simulink model "SegOrdem"  (R2015a)
settings: Solver=ode45  StartTime=0.0  StopTime=60  FixedStep=0.00001  RelTol=1e-5
settings Model: Creator=user  LastModifiedBy=user
settings SolverCC: ZeroCrossAlgorithm=Adaptive
settings DebuggingCC: UnderspecifiedInitializationDetection=Classic

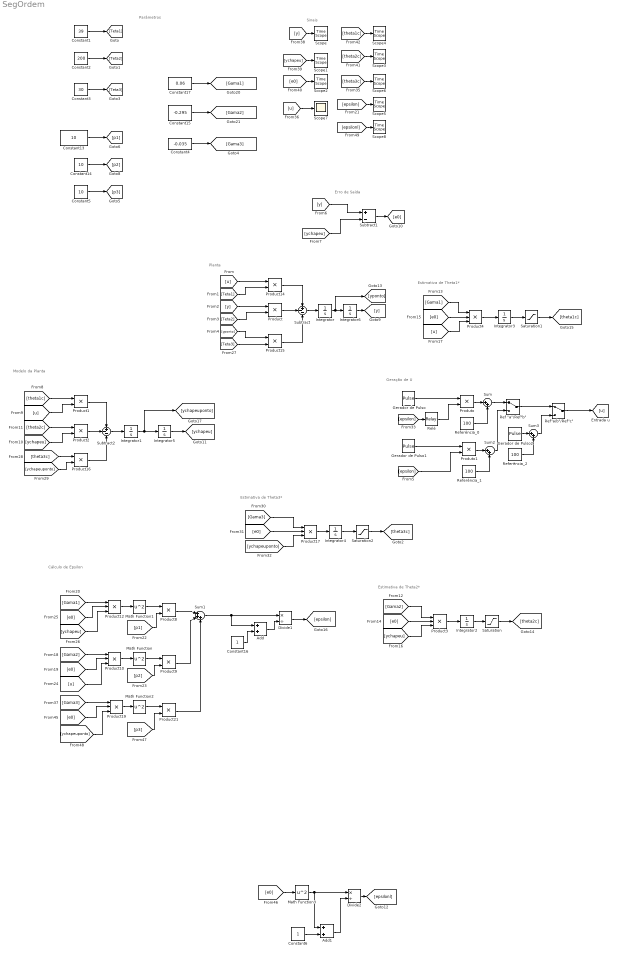
== system SegOrdem ==
  note: Cálculo de Epsilon
  note: Estimativa de Theta1*
  note: Estimativa de Theta2*
  note: Modelo da Planta
  note: Erro de Saída
  note: Parâmetros
  note: Sinais
  note: Estimativa de Theta3*
  note: Planta
  note: Geração de U
  Add : Sum  AccumDataTypeStr=double
  Add1 : Sum  AccumDataTypeStr=double
  Constant1 : Constant  Value=39
  Constant13 : Constant  Value=10
  Constant14 : Constant  Value=10
  Constant15 : Constant  Value=-0.295
  Constant16 : Constant
  Constant17 : Constant  Value=0.06
  Constant2 : Constant  Value=200
  Constant3 : Constant  Value=30
  Constant4 : Constant  Value=-0.035
  Constant5 : Constant  Value=10
  Constant6 : Constant
  Divide1 : Product  Inputs=*/  OutDataTypeStr=double
  Divide2 : Product  Inputs=*/  OutDataTypeStr=double
  Gerador de Pulso : DiscretePulseGenerator  PulseType=Time based  Amplitude=100  Period=0.5  PulseWidth=50
  Gerador de Pulso1 : DiscretePulseGenerator  PulseType=Time based  Amplitude=100  Period=0.5  PulseWidth=50
  Gerador de Pulso2 : DiscretePulseGenerator  PulseType=Time based  Amplitude=100  Period=0.5  PulseWidth=50
  Integrator{,1,5..6} (4 alike) : Integrator
  Integrator2 : Integrator  InitialCondition=70
  Integrator3 : Integrator  InitialCondition=80
  Integrator4 : Integrator  InitialCondition=5
  Math Function{,1..3} (4 alike) : Math  Operator=square  SaturateOnIntegerOverflow=on
  Product{,1..2,8..9,14..16,21} (9 alike) : Product
  Product{3..4,10,12,17,19} (6 alike) : Product  Inputs=3
  Produto : Product
  Produto1 : Product
  "Ref \"a\"/Ref\"b\"" : ManualSwitch
  "Ref\"a/b\"/Ref\"c\"" : ManualSwitch
  Referência_0 : Constant  Value=100
  Referência_1 : Constant  Value=100
  Referência_2 : Constant  Value=100
  Relé : Relay  OnSwitchValue=0.5  OffSwitchValue=0.5
  Saturation : Saturate  UpperLimit=50000  LowerLimit=0
  Saturation1 : Saturate  UpperLimit=300000  LowerLimit=0
  Saturation2 : Saturate  UpperLimit=30000  LowerLimit=0
  Scope{,1..6,8} (8 alike) : TimeScope
  Scope7 : Scope
      settings: YMin=-12  YMax=12  SaveName=ScopeData5  SampleInput=on
  Subtract : Sum  Inputs=+--
  Subtract1 : Sum  Inputs=+-
  Subtract2 : Sum  Inputs=+--
  Sum : Sum  Inputs=|++
  Sum1 : Sum  Inputs=|+++
  Sum2 : Sum  Inputs=|++
  Sum3 : Sum  Inputs=|++
  wires:
  [Teta1] -> Product14/2
  [Teta2] -> Product/2
  Product/1 -> Subtract/2
  Product14/1 -> Subtract/1
  Subtract/1 -> Integrator/1
  [y] -> Product/1
  [u] -> Product14/1
  [y] -> Subtract1/1
  [ychapeu] -> Subtract1/2
  Subtract1/1 -> [e0]
  Constant1/1 -> [Teta1]
  Constant2/1 -> [Teta2]
  Product1/1 -> Subtract2/1
  Subtract2/1 -> Integrator1/1
  Product2/1 -> Subtract2/2
  [theta2c] -> Product2/1
  [u] -> Product1/2
  [theta1c] -> Product1/1
  [e0] -> Product3/2
  [Gama2] -> Product3/1
  [Gama1] -> Product4/1
  [e0] -> Product4/2
  [ychapeu] -> Product3/3
  [u] -> Product4/3
  Product3/1 -> Integrator2/1
  Product4/1 -> Integrator3/1
  Integrator3/1 -> Saturation1/1
  Integrator2/1 -> Saturation/1
  Product10/1 -> Math Function/1
  Product12/1 -> Math Function1/1
  Math Function1/1 -> Product8/1
  Math Function/1 -> Product9/1
  [p1] -> Product8/2
  [p2] -> Product9/2
  Product9/1 -> Sum1/2
  Product8/1 -> Sum1/1
  Constant13/1 -> [p1]
  Constant14/1 -> [p2]
  [y] -> Scope/1
  [ychapeu] -> Scope1/1
  [e0] -> Scope2/1
  [theta2c] -> Scope3/1
  [theta1c] -> Scope4/1
  Constant17/1 -> [Gama1]
  Constant15/1 -> [Gama2]
  Add/1 -> Divide1/2
  Constant16/1 -> Add/2
  Sum1/1 -> Add/1, Divide1/1
  Saturation/1 -> [theta2c]
  Saturation1/1 -> [theta1c]
  [Gama2] -> Product10/1
  [e0] -> Product10/2
  [u] -> Product10/3
  [e0] -> Product12/2
  [Gama1] -> Product12/1
  [ychapeu] -> Product12/3
  [epsilon] -> Scope5/1
  [yponto] -> Product15/1
  [Teta3] -> Product15/2
  Product15/1 -> Subtract/3
  [ychapeuponto] -> Product16/2
  [theta3c] -> Product16/1
  Product16/1 -> Subtract2/3
  [Gama3] -> Product17/1
  [e0] -> Product17/2
  [ychapeuponto] -> Product17/3
  Product17/1 -> Integrator4/1
  Integrator4/1 -> Saturation2/1
  Saturation2/1 -> [theta3c]
  Constant3/1 -> [Teta3]
  Constant4/1 -> [Gama3]
  Constant5/1 -> [p3]
  Integrator5/1 -> [ychapeu]
  Integrator6/1 -> [y]
  Integrator/1 -> [yponto], Integrator6/1
  Integrator1/1 -> Integrator5/1, [ychapeuponto]
  [theta3c] -> Scope6/1
  Divide1/1 -> [epsilon]
  [u] -> Scope7/1
  Product19/1 -> Math Function2/1
  Math Function2/1 -> Product21/1
  [p3] -> Product21/2
  [Gama3] -> Product19/1
  [e0] -> Product19/2
  [ychapeuponto] -> Product19/3
  Product21/1 -> Sum1/3
  [e0] -> Math Function3/1
  Math Function3/1 -> Divide2/1, Add1/1
  Constant6/1 -> Add1/2
  Add1/1 -> Divide2/2
  Divide2/1 -> [epsilonl]
  [epsilonl] -> Scope8/1
  [ychapeu] -> Product2/2
  Referência_0/1 -> Sum/2
  Sum/1 -> "Ref \"a\"/Ref\"b\""/1
  Produto/1 -> Sum/1
  Gerador de Pulso/1 -> Produto/1
  [epsilon] -> Relé/1
  Relé/1 -> Produto/2
  "Ref \"a\"/Ref\"b\""/1 -> "Ref\"a/b\"/Ref\"c\""/1
  Referência_1/1 -> Sum2/2
  Produto1/1 -> Sum2/1
  Gerador de Pulso1/1 -> Produto1/1
  [epsilon] -> Produto1/2
  Sum2/1 -> "Ref \"a\"/Ref\"b\""/2
  "Ref\"a/b\"/Ref\"c\""/1 -> [u]
  Sum3/1 -> "Ref\"a/b\"/Ref\"c\""/2
  Gerador de Pulso2/1 -> Sum3/1
  Referência_2/1 -> Sum3/2
